simulink model "Erdorbits"  (Simulink 7.9)
settings: Solver=ode45  StartTime=0.0  StopTime=10.0  RelTol=1e-3
settings Model: Creator=karo  LastModifiedBy=karo

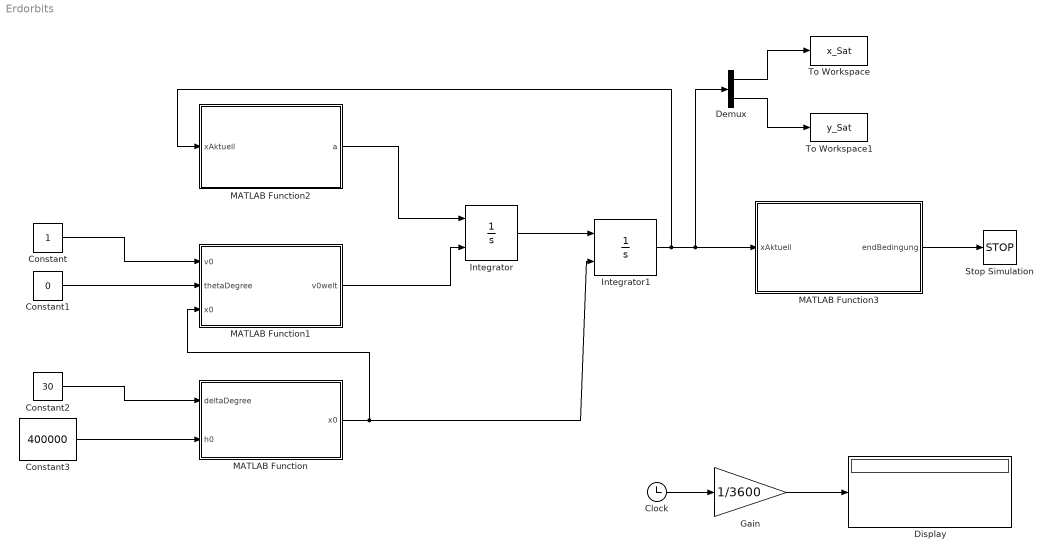
== system Erdorbits ==
  Clock : Clock
  Constant : Constant
  Constant1 : Constant  Value=0
  Constant2 : Constant  Value=30
  Constant3 : Constant  Value=400000
  Demux : Demux  Outputs=2
  Display : Display
  Gain : Gain  Gain=1/3600
  Integrator : Integrator  InitialConditionSource=external
  Integrator1 : Integrator  InitialConditionSource=external
  MATLAB Function : MATLAB Function  TreatAsAtomicUnit=on
  MATLAB Function1 : MATLAB Function  TreatAsAtomicUnit=on
  MATLAB Function2 : MATLAB Function  TreatAsAtomicUnit=on
  MATLAB Function3 : MATLAB Function  TreatAsAtomicUnit=on
  Stop Simulation : Stop
  To Workspace : ToWorkspace  VariableName=x_Sat  SampleTime=-1  SaveFormat=Timeseries
  To Workspace1 : ToWorkspace  VariableName=y_Sat  SampleTime=-1  SaveFormat=Timeseries
  wires:
  MATLAB Function1/1(v0welt) -> Integrator/2
  MATLAB Function2/1(a) -> Integrator/1
  Integrator/1 -> Integrator1/1
  Integrator1/1 -> MATLAB Function2/1(xAktuell), MATLAB Function3/1(xAktuell), Demux/1
  MATLAB Function/1(x0) -> Integrator1/2, MATLAB Function1/3(x0)
  MATLAB Function3/1(endBedingung) -> Stop Simulation/1
  Constant3/1 -> MATLAB Function/2(h0)
  Constant2/1 -> MATLAB Function/1(deltaDegree)
  Constant1/1 -> MATLAB Function1/2(thetaDegree)
  Constant/1 -> MATLAB Function1/1(v0)
  Clock/1 -> Gain/1
  Gain/1 -> Display/1
  Demux/2 -> To Workspace1/1
  Demux/1 -> To Workspace/1

== matlab function MATLAB Function1 ==
  data: v0 input double; v0welt output double; thetaDegree input double; x0 input double
function v0welt = vStart(v0, thetaDegree, x0)
%#codegen

% v0 - Startgeschwindigkeit
% thetaDegree Winket theta in Grad
% x0 STartposition

nE = x0 / norm(x0);     % Einheitsvektor in Normalrichtung für x0
tE = [nE(2) ; -nE(1)];  % Einheitvektor in Tangentialrichtung für x0

vt = cosd(thetaDegree) * v0;    % Tangentialkomponente für v0
vn = sind(thetaDegree) * v0;    % Normalkomponente für v0

v0welt = tE * vt + nE * vn;     % Geschwindigkeitsvektor

== matlab function MATLAB Function ==
  data: deltaDegree input double; x0 output double; h0 input double
function x0 = Startposition(deltaDegree, h0)
%#codegen
r = 6378000;   % Erdradius [m]
h = r + h0;    % Hypothenuse
x0 = [cosd(deltaDegree) * h ; sind(deltaDegree) * h ];

== matlab function MATLAB Function2 ==
  data: xAktuell input double; a output double
function a = Beschleunigung(xAktuell)
%#codegen

xE = xAktuell / norm(xAktuell);   % Einheiitsvektor für xAktuell
eSE = xE * (-1);    % Einheitsvektor vom Satelliten zu Erde - umgekehrte Richtung zu xE

r = norm(xAktuell); % Abstand von Erdmitte zum Satellit

mE = 5.9736 * 10^24;    % Erdmasse in [kg]
G = 66.743 * 10^-12;    % Gravitationskonstante in [m^3/kg*s^2]

a = G * mE / r^2 * eSE; % Beschleunigung

== matlab function MATLAB Function3 ==
  data: xAktuell input double; endBedingung output double
function endBedingung = Kontakt(xAktuell)
%#codegen

rErde = 6378000;
xAbstand = norm(xAktuell);

if (xAbstand > rErde) 
    endBedingung = 0;
else
    endBedingung = 1;
end
